simulink model "Verifica_EIG_11032026_es"  (R2025b)
settings: Solver=VariableStepAuto  StartTime=0.0  StopTime=10.0  RelTol=1e-3
undefined symbols (not defined in the file): A, B, K_eig, m, N, n, r, x0_eig
settings Model: Creator=salvo  LastModifiedBy=salvo

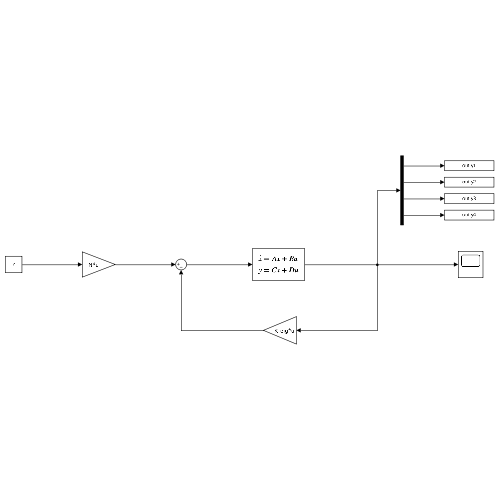
[thumbnail: Simulink's stored preview of the top-level diagram]
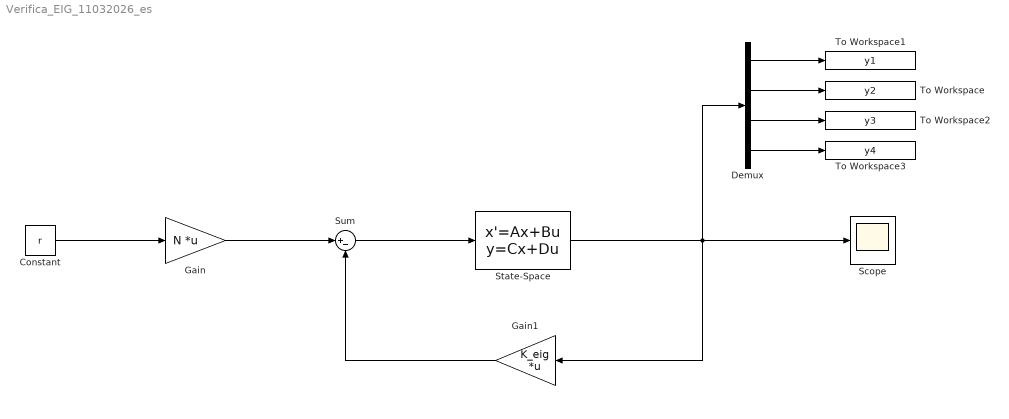
== system Verifica_EIG_11032026_es ==
  Constant : Constant  Value=r
  Demux : Demux
  Gain : Gain  Gain=N  Multiplication=Matrix(K*u)
  Gain1 : Gain  Gain=K_eig  Multiplication=Matrix(K*u)
  Scope : Scope
      settings: ActiveDisplayYMinimum=-1.6733586877925997  ActiveDisplayYMaximum=2.7085781495442709
  State-Space : StateSpace  A=A  B=B  C=eye(n)  D=zeros(n,m)  InitialCondition=x0_eig
  Sum : Sum  Inputs=|+-
  To Workspace : ToWorkspace  VariableName=y2  SaveFormat=Timeseries  SampleTime=-1
  To Workspace1 : ToWorkspace  VariableName=y1  SaveFormat=Timeseries  SampleTime=-1
  To Workspace2 : ToWorkspace  VariableName=y3  SaveFormat=Timeseries  SampleTime=-1
  To Workspace3 : ToWorkspace  VariableName=y4  SaveFormat=Timeseries  SampleTime=-1
  wires:
  Constant/1 -> Gain/1
  Gain1/1 -> Sum/2
  Gain/1 -> Sum/1
  Sum/1 -> State-Space/1
  State-Space/1 -> Demux/1, Gain1/1, Scope/1
  Demux/2 -> To Workspace/1
  Demux/1 -> To Workspace1/1
  Demux/3 -> To Workspace2/1
  Demux/4 -> To Workspace3/1
